simulink subsystem "HV_Battery"  (R2022a)
settings: Solver=VariableStepAuto  StartTime=0.0  StopTime=2474  RelTol=1e-3
model mask{batt_energy=53.5, batt_nominal_voltage=800, coolant_lpm=33.33, coolant_quantity=10, coolant_inlet_temp=25, cell_ambient_temp=35, peak_dischg_c_rate=2, peak_chg_c_rate=2, cont_dischg_c_rate=1, cont_chg_c_rate=1, peak_time=30, peak_time_dischg=0.9, batt_init_soc=0.9}
  mask prompts: batt_energy "Enter the Battery Energy [in kWh]"; batt_nominal_voltage "Enter Battery Nominal Voltage [in V]"; coolant_lpm "Enter Coolant Flow Rate [in LPM]"; coolant_quantity "Enter Coolant Quantity in system [in gallons]"; coolant_inlet_temp "Enter Coolant Initial Inlet Temperature [in Celcius]"; cell_ambient_temp "Enter Local Ambient Cell Temperature [in Celcius]"; peak_dischg_c_rate "Enter Peak Discharge C Rate"; peak_chg_c_rate "Enter Peak Charge C Rate"; cont_dischg_c_rate "Enter Continuous Discharge C Rate"; cont_chg_c_rate "Enter Continuous Charge C Rate"; peak_time "Enter Maximum Duration for Peak Charging C Rate [in seconds]"; peak_time_dischg "Enter Maximum Duration for Peak Discharging C Rate [in seconds]"; batt_init_soc "Enter Initial Battery SOC [0 to 1]"
undefined symbols (not defined in the file or in its folder): batt, cell_Ah, cell_col_eff, cell_cp, cell_eff_area, cell_heat_trans_coeff, cell_mass, cont_chg_current, cont_dischg_current, coolant_cp, coolant_mass, coolant_mass_dot, num_bricks_parallel_in_one_module, num_bricks_series_in_one_module, num_cell_parallel_in_one_brick, num_cell_series_in_one_brick, num_module_Parallel, num_module_Series, peak_chg_current, peak_dischg_current, Total_num_cells
libraries: simulink x18, aerolibconvert2 x3, autolibshared x1
settings Model: DefaultTestHarness=HV_Battery_Harness2  Creator=aak  LastModifiedBy=saumilj

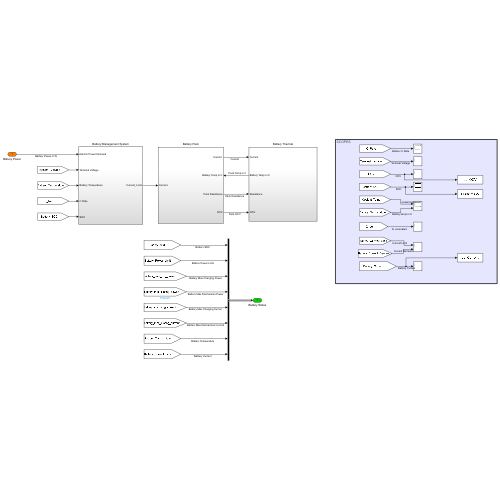
[thumbnail: Simulink's stored preview of the top-level diagram]
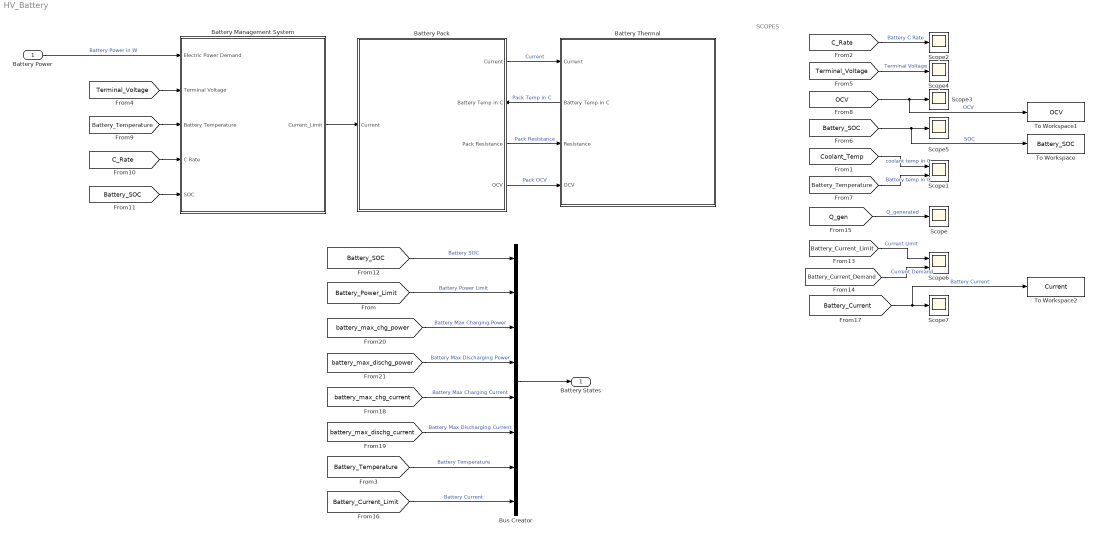
== system HV_Battery ==
  note: SCOPES
  Battery Power : Inport
  Battery Management System : Subsystem
  Battery Pack : Subsystem
      settings: PortSchema="{\"entries\":[{\"content\":{\"sides\":[{\"content\":{\"connectorIds\":[\"In1\"]},\"type\":\"ConnectorPlacement.EquallySpacedRectSide\",\"uuid\":\"b9545a5c-edfc-42ef-81ab-9f23645d84e0\"},{\"content\":{\"connectorIds\":[\"Out1\",\"In2\",\"Out2\",\"Out3\"],\"side\":\"RIGHT\"},\"type\":\"ConnectorPlacement.EquallySpacedRectSide\",\"uuid\":\"40135f2d-ea88-44e9-aecc-89357aa4ea88\"},{\"content\":{\"connectorIds\":[],\"side\":\"TOP\"},\"type\":\"ConnectorPlacement.EquallySpacedRectSide\",\"uuid\":\"2e3e458a-5c5e-47fb-9bfa-05c4f097828d\"},{\"content\":{\"connectorIds\":[],\"side\":\"BOTTOM\"},\"type\":\"ConnectorPlacement.EquallySpacedRectSide\",\"uuid\":\"704f8b5a-b8e4-4dd9-930b-8f21277b1215\"}]},\"type\":\"ConnectorPlacement.EquallySpacedConnector\",\"uuid\":\"37de8f39-e745-4310-bdfe-a8e78e320ee8\"}],\"packageUris\":[\"http://schema.mathworks.com/mf0/Connector/R2020b\"],\"version\":\"1.0\"}"
  Battery Thermal : Subsystem
      settings: PortSchema="{\"entries\":[{\"content\":{\"sides\":[{\"content\":{\"connectorIds\":[\"In1\",\"Out1\",\"In2\",\"In3\"]},\"type\":\"ConnectorPlacement.EquallySpacedRectSide\",\"uuid\":\"af3b2aec-6ad7-445b-b1a0-7265fbd6b2ee\"},{\"content\":{\"connectorIds\":[],\"side\":\"RIGHT\"},\"type\":\"ConnectorPlacement.EquallySpacedRectSide\",\"uuid\":\"a27c7f15-5848-4e0f-a52c-5f856bed419f\"},{\"content\":{\"connectorIds\":[],\"side\":\"TOP\"},\"type\":\"ConnectorPlacement.EquallySpacedRectSide\",\"uuid\":\"1e997449-128f-4f3b-ad87-015e7077aed3\"}]},\"type\":\"ConnectorPlacement.EquallySpacedConnector\",\"uuid\":\"f88aa6e9-d781-4b9c-928f-406822c5ea22\"}],\"packageUris\":[\"http://schema.mathworks.com/mf0/Connector/R2020b\"],\"version\":\"1.0\"}"
  Bus Creator : BusCreator  Inputs=8
  Scope{,2..5,7} (6 alike) : Scope
  Scope1 : Scope  NumInputPorts=2
  Scope6 : Scope  NumInputPorts=2
  To Workspace : ToWorkspace  VariableName=Battery_SOC  SampleTime=-1
  To Workspace1 : ToWorkspace  VariableName=OCV  SampleTime=-1
  To Workspace2 : ToWorkspace  VariableName=Current  SampleTime=-1
  Battery States : Outport
  wires:
  Battery Pack/1("Current ") -> Battery Thermal/1("Current ")  "Current"
  Battery Power/1 -> Battery Management System/1(Electric Power Demand)  "Battery Power in W"
  [Battery_SOC] -> To Workspace/1, Scope5/1  "SOC"
  [OCV] -> To Workspace1/1, Scope3/1  "OCV"
  Battery Thermal/1(Battery Temp in C) -> Battery Pack/2(Battery Temp in C)  "Pack Temp in C"
  [Battery_SOC] -> Battery Management System/5(SOC)
  [Battery_Temperature] -> Scope1/2  "Battery temp in C"
  Battery Management System/1(Current_Limit) -> Battery Pack/1(Current)
  [Terminal_Voltage] -> Battery Management System/2(Terminal Voltage)
  [Battery_SOC] -> Bus Creator/1  "Battery SOC"
  [C_Rate] -> Scope2/1  "Battery C Rate"
  [Battery_Temperature] -> Battery Management System/3(Battery Temperature)
  [Coolant_Temp] -> Scope1/1  "coolant temp in C"
  [Terminal_Voltage] -> Scope4/1  "Terminal Voltage"
  Bus Creator/1 -> Battery States/1
  Battery Pack/2(" Pack Resistance") -> Battery Thermal/2(Resistance)  "Pack Resistance"
  Battery Pack/3(OCV) -> Battery Thermal/3(OCV)  "Pack OCV"
  [C_Rate] -> Battery Management System/4(C Rate)
  [Battery_Power_Limit] -> Bus Creator/2  "Battery Power Limit"
  [Battery_Current_Limit] -> Scope6/1  "Current Limit"
  [Battery_Current_Demand] -> Scope6/2  "Current Demand"
  [Q_gen] -> Scope/1  "Q_generated"
  [Battery_Current] -> To Workspace2/1, Scope7/1  "Battery Current"
  [battery_max_chg_current] -> Bus Creator/5  "Battery Max Charging Current"
  [battery_max_dischg_current] -> Bus Creator/6  "Battery Max Discharging Current"
  [Battery_Temperature] -> Bus Creator/7  "Battery Temperature"
  [Battery_Current_Limit] -> Bus Creator/8  "Battery Current"
  [battery_max_dischg_power] -> Bus Creator/4  "Battery Max Discharging Power"
  [battery_max_chg_power] -> Bus Creator/3  "Battery Max Charging Power"

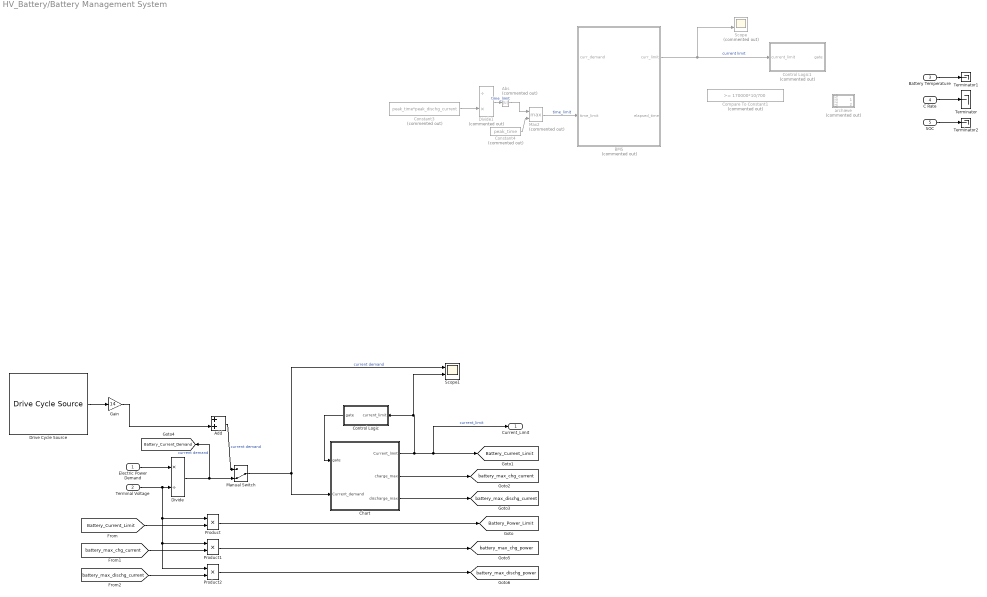
== system HV_Battery/Battery Management System ==
  Electric Power Demand : Inport
  Terminal Voltage : Inport  Port=2
  Battery Temperature : Inport  Port=3
  C Rate : Inport  Port=4
  SOC : Inport  Port=5
  Abs : Abs  Commented=on  SaturateOnIntegerOverflow=off
  Add : Sum
  BMS : Stateflow chart  Commented=on  TreatAsAtomicUnit=on
  Chart : Stateflow chart  TreatAsAtomicUnit=on
      settings: PortSchema="{\"entries\":[{\"content\":{\"sides\":[{\"content\":{\"connectorIds\":[\"In2\",\"In1\"]},\"type\":\"ConnectorPlacement.EquallySpacedRectSide\",\"uuid\":\"61e53cb5-f277-4f3d-99e4-fd5a81de5d3f\"},{\"content\":{\"connectorIds\":[\"Out1\",\"Out2\",\"Out3\"],\"side\":\"RIGHT\"},\"type\":\"ConnectorPlacement.EquallySpacedRectSide\",\"uuid\":\"0e0f51c4-d227-4234-809c-9980418e03b4\"},{\"content\":{\"connectorIds\":[],\"side\":\"TOP\"},\"type\":\"ConnectorPlacement.EquallySpacedRectSide\",\"uuid\":\"31baac4d-e034-4979-aab1-cd5457b5efab\"}]},\"type\":\"ConnectorPlacement.EquallySpacedConnector\",\"uuid\":\"6907569d-9725-4403-be47-b0224ef335f3\"}],\"packageUris\":[\"http://schema.mathworks.com/mf0/Connector/R2020b\"],\"version\":\"1.0\"}"
  Compare To Constant1 : simulink/Logic and Bit Operations/Compare To Constant  Commented=on  relop=>=  const=170000*10/700  OutDataTypeStr=boolean
  Constant3 : Constant  Commented=on  Value=peak_time*peak_dischg_current
  Constant4 : Constant  Commented=on  Value=peak_time
  Control Logic : Subsystem
      settings: PortSchema="{\"entries\":[{\"content\":{\"sides\":[{\"content\":{\"connectorIds\":[\"Out1\"]},\"type\":\"ConnectorPlacement.EquallySpacedRectSide\",\"uuid\":\"375a58bc-16a4-4cbe-8416-d0abc0116f23\"},{\"content\":{\"connectorIds\":[\"In1\"],\"side\":\"RIGHT\"},\"type\":\"ConnectorPlacement.EquallySpacedRectSide\",\"uuid\":\"b00af4b7-7940-47c4-950c-bf6d404947a6\"},{\"content\":{\"connectorIds\":[],\"side\":\"TOP\"},\"type\":\"ConnectorPlacement.EquallySpacedRectSide\",\"uuid\":\"5f8d3327-63b2-477e-9ddb-4def616de5d9\"}]},\"type\":\"ConnectorPlacement.EquallySpacedConnector\",\"uuid\":\"dfdcbaa4-409c-473f-908d-88d904123078\"}],\"packageUris\":[\"http://schema.mathworks.com/mf0/Connector/R2020b\"],\"version\":\"1.0\"}"
  Control Logic1 : Subsystem  Commented=on
  Divide : Product  Inputs=*/
  Divide1 : Product  Commented=on  Inputs=/*
  Drive Cycle Source : autolibshared/Drive Cycle Source  cycleVar=FTP75  fileVar=cycleFTP75.mat  tfinal="2474  seconds, Cyclic"  cycleRepeat=on  outAccPort=off  outGearPort=off  gearList=No gear data  t_wot1=5  xdot_woto=0  xdot_wot1=30  t_wot2=20  xdot_wot2=0  t_wotend=30  srcUnit=m/s  outUnit=m/s  srcAccUnit=m/s/s  outAccUnit=m/s^2  dt=1  aMode=1  faultOption=off  velBnd=2  velBndUnit=mph  inUnit=m/s  timeBnd=1  failOption=off  stopSim=off  maxFaultCnt=10  maxFaultTime=2  maxTotFaultTime=15  traceOption=off  dtTrace=1  traceWindow=10  lastDCname=FTP75  lastOutUnit=mph  lastDT=1  lastTB=1  lastSB=2  forceCalcBound=off
      settings: SourceProductBaseCode=PW,DR,MT,VE
  Gain : Gain  Gain=14
  Manual Switch : ManualSwitch  CurrentSetting=0
  Max2 : MinMax  Commented=on  Function=max  Inputs=2
  Product : Product
  Product1 : Product
  Product2 : Product
  Scope : Scope  Commented=on  NumInputPorts=2
  Scope1 : Scope  NumInputPorts=2
  Terminator : Terminator
  Terminator1 : Terminator
  Terminator2 : Terminator
  archieve : Subsystem  Commented=on
  Current_Limit : Outport
  tag scope: Battery_Current_Demand=global, Battery_Current_Limit=global, Battery_Power_Limit=global, battery_max_chg_current=global, battery_max_chg_power=global, battery_max_dischg_current=global, battery_max_dischg_power=global
  wires:
  [battery_max_dischg_current] -> Product2/2
  Product2/1 -> [battery_max_dischg_power]
  Product1/1 -> [battery_max_chg_power]
  [battery_max_chg_current] -> Product1/2
  Control Logic/1(gate) -> Chart/2(gate)
  Electric Power Demand/1 -> Divide/1
  Drive Cycle Source/1 -> Gain/1
  Product/1 -> [Battery_Power_Limit]
  [Battery_Current_Limit] -> Product/2
  Manual Switch/1 -> Chart/1(Current_demand), Scope1/1  "current demand"
  Add/1 -> Manual Switch/1  "current demand"
  Gain/1 -> Add/2
  Chart/1(Current_limit) -> Scope1/2, Control Logic/1(current_limit), Current_Limit/1, [Battery_Current_Limit]  "current_limit"
  BMS/1(curr_limit) -> Control Logic1/1(current_limit), Scope/2  "current limit"
  Abs/1 -> Max2/1
  Constant4/1 -> Max2/2
  Max2/1 -> BMS/2(time_limit)  "time_limit"
  Divide/1 -> Manual Switch/2, [Battery_Current_Demand]  "current demand"
  Terminal Voltage/1 -> Divide/2, Product/1, Product1/1, Product2/1
  C Rate/1 -> Terminator/1
  Battery Temperature/1 -> Terminator1/1
  SOC/1 -> Terminator2/1
  Divide1/1 -> Abs/1  "time_limit"
  Constant3/1 -> Divide1/2
  Chart/2(charge_max) -> [battery_max_chg_current]
  Chart/3(discharge_max) -> [battery_max_dischg_current]

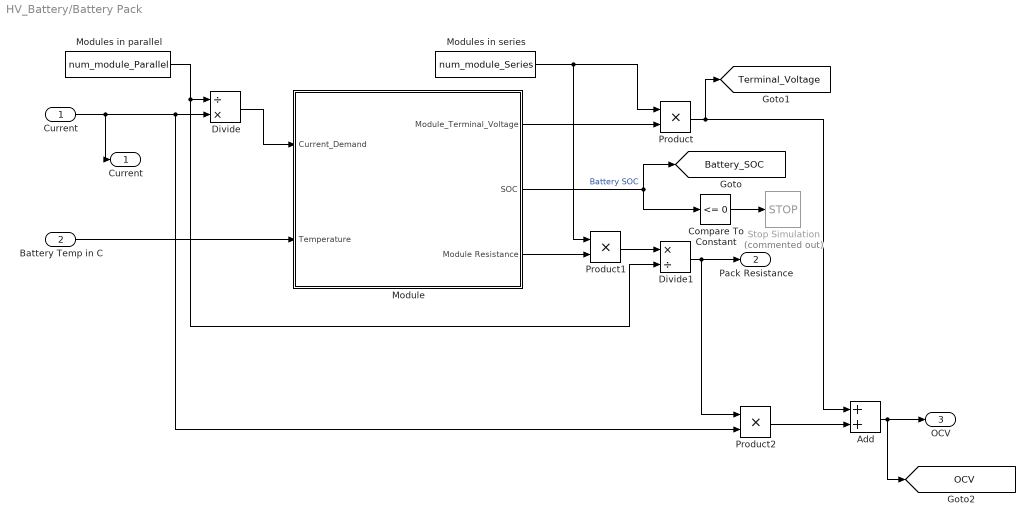
== system HV_Battery/Battery Pack ==
  Current : Inport
  Battery Temp in C : Inport  Port=2
  Add : Sum
  Compare To Constant : simulink/Logic and Bit Operations/Compare To Constant  relop=<=  const=0  OutDataTypeStr=boolean
  Divide : Product  Inputs=/*
  Divide1 : Product  Inputs=*/
  Module : Subsystem
  Modules in parallel : Constant  Value=num_module_Parallel
  Modules in series : Constant  Value=num_module_Series
  Product : Product
  Product1 : Product
  Product2 : Product
  Stop Simulation : Stop  Commented=on
  "Current " : Outport
  " Pack Resistance" : Outport  Port=2
  OCV : Outport  Port=3
  tag scope: Battery_SOC=global, OCV=global, Terminal_Voltage=global
  wires:
  Module/2(" SOC") -> Compare To Constant/1, [Battery_SOC]  "Battery SOC"
  Compare To Constant/1 -> Stop Simulation/1
  Divide/1 -> Module/1(Current_Demand)
  Module/1(Module_Terminal_Voltage) -> Product/2
  Product/1 -> [Terminal_Voltage], Add/1
  Divide1/1 -> Product2/1, " Pack Resistance"/1
  Modules in series/1 -> Product/1, Product1/1
  Product1/1 -> Divide1/1
  Module/3(" Module Resistance") -> Product1/2
  Modules in parallel/1 -> Divide/1, Divide1/2
  Battery Temp in C/1 -> Module/2(Temperature)
  Product2/1 -> Add/2
  Add/1 -> OCV/1, [OCV]
  Current/1 -> Product2/2, Divide/2, "Current "/1

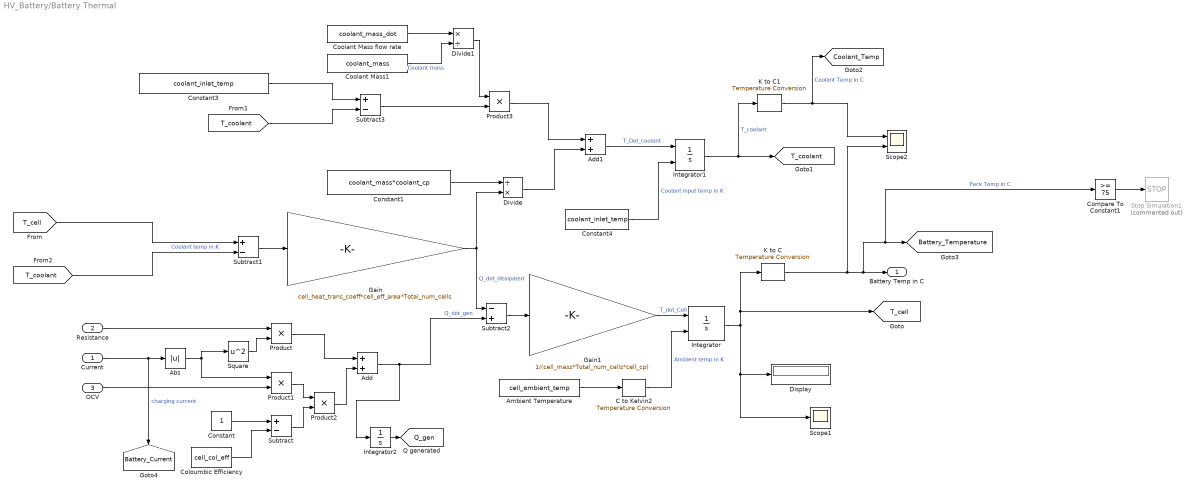
== system HV_Battery/Battery Thermal ==
  "Current " : Inport
  Resistance : Inport  Port=2
  OCV : Inport  Port=3
  Abs : Abs  SaturateOnIntegerOverflow=off
  Add : Sum
  Add1 : Sum
  Ambient Temperature : Constant  Value=cell_ambient_temp
  C to Kelvin2 : aerolibconvert2/Temperature Conversion  IU=C  OU=K
      settings: SourceProductBaseCode=AE
  Coloumbic Efficiency : Constant  Value=cell_col_eff
  Compare To Constant1 : simulink/Logic and Bit Operations/Compare To Constant  relop=>=  const=75  OutDataTypeStr=boolean
  Constant : Constant
  Constant1 : Constant  Value=coolant_mass*coolant_cp
  Constant3 : Constant  Value=coolant_inlet_temp
  Constant4 : Constant  Value=coolant_inlet_temp
  Coolant Mass flow rate : Constant  Value=coolant_mass_dot
  Coolant Mass1 : Constant  Value=coolant_mass
  Display : Display
  Divide : Product  Inputs=/*
  Divide1 : Product  Inputs=*/
  Gain : Gain  Gain=cell_heat_trans_coeff*cell_eff_area*Total_num_cells
  Gain1 : Gain  Gain=1/(cell_mass*Total_num_cells*cell_cp)
  Integrator : Integrator  InitialConditionSource=external  InitialCondition=273+25
  Integrator1 : Integrator  InitialConditionSource=external
  Integrator2 : Integrator
  K to C : aerolibconvert2/Temperature Conversion  IU=K  OU=C
      settings: SourceProductBaseCode=AE
  K to C1 : aerolibconvert2/Temperature Conversion  IU=K  OU=C
      settings: SourceProductBaseCode=AE
  Product{,1..3} (4 alike) : Product
  Scope1 : Scope
  Scope2 : Scope  NumInputPorts=2
  Square : Math  Operator=square
  Stop Simulation1 : Stop  Commented=on
  Subtract : Sum  Inputs=+-
  Subtract1 : Sum  Inputs=+-
  Subtract2 : Sum  Inputs=-+
  Subtract3 : Sum  Inputs=+-
  Battery Temp in C : Outport
  tag scope: Battery_Current=global, Battery_Temperature=global, Coolant_Temp=global, Q_gen=global, T_cell=global, T_coolant=global
  wires:
  K to C/1 -> Scope2/2, Battery Temp in C/1, [Battery_Temperature], Compare To Constant1/1  "Pack Temp in C"
  Compare To Constant1/1 -> Stop Simulation1/1
  Resistance/1 -> Product/1
  Square/1 -> Product/2
  OCV/1 -> Product1/2
  Constant/1 -> Subtract/1
  Coloumbic Efficiency/1 -> Subtract/2
  Product1/1 -> Product2/1
  Subtract/1 -> Product2/2
  Product/1 -> Add/1
  Product2/1 -> Add/2
  Add/1 -> Integrator2/1, Subtract2/2  "Q_dot_gen"
  [T_coolant] -> Subtract1/2  "Coolant temp in K"
  Subtract1/1 -> Gain/1
  Gain1/1 -> Integrator/1  "T_dot_Cell"
  Integrator/1 -> Display/1, Scope1/1, K to C/1, [T_cell]
  [T_cell] -> Subtract1/1
  Subtract2/1 -> Gain1/1
  Gain/1 -> Subtract2/1, Divide/2  "Q_dot_dissipated"
  Ambient Temperature/1 -> C to Kelvin2/1
  C to Kelvin2/1 -> Integrator/2  "Ambient temp in K"
  Constant1/1 -> Divide/1
  Divide/1 -> Add1/2
  Constant3/1 -> Subtract3/1
  [T_coolant] -> Subtract3/2
  Subtract3/1 -> Product3/2
  Product3/1 -> Add1/1
  Add1/1 -> Integrator1/1  "T_Dot_coolant"
  Integrator1/1 -> K to C1/1, [T_coolant]  "T_coolant"
  "Current "/1 -> [Battery_Current], Abs/1  "charging current"
  Coolant Mass flow rate/1 -> Divide1/1
  Divide1/1 -> Product3/1
  Coolant Mass1/1 -> Divide1/2  "Coolant mass"
  Constant4/1 -> Integrator1/2  "Coolant input temp in K"
  K to C1/1 -> [Coolant_Temp], Scope2/1  "Coolant Temp in C"
  Abs/1 -> Square/1, Product1/1
  Integrator2/1 -> [Q_gen]

== system HV_Battery/Battery Management System/Control Logic ==
  current_limit : Inport
  Charging : Subsystem
  Discharging : Subsystem
  Switch : Switch  Criteria=u2 > Threshold  SaturateOnIntegerOverflow=off  InputSameDT=off
  gate : Outport
  wires:
  current_limit/1 -> Discharging/1(current limit), Switch/2, Charging/1(current limit)
  Charging/1(charging gate) -> Switch/3, gate/1
  Discharging/1(discharging gate) -> Switch/1

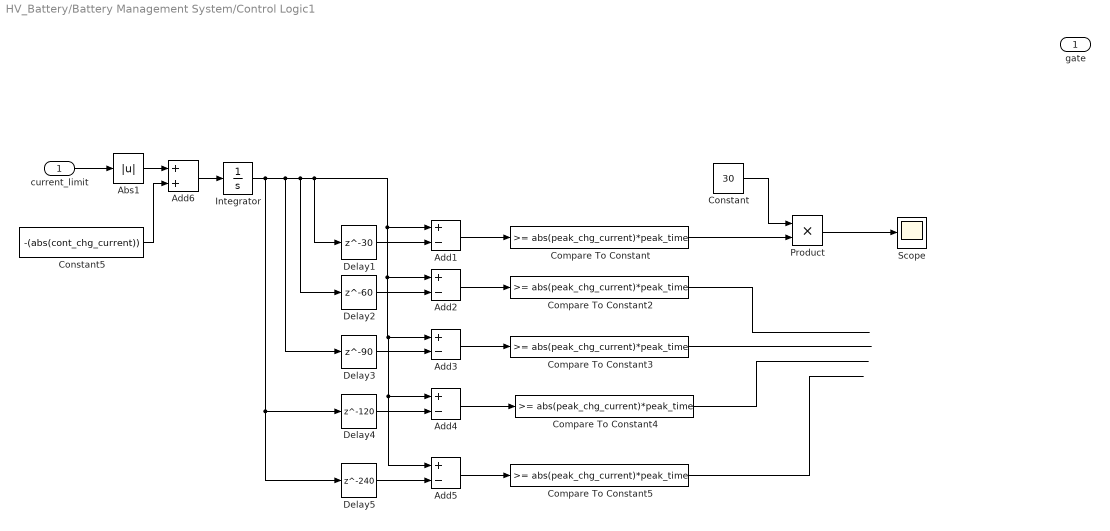
== system HV_Battery/Battery Management System/Control Logic1 ==
  current_limit : Inport
  Abs1 : Abs  SaturateOnIntegerOverflow=off
  Add{1..5} (5 alike) : Sum  Inputs=+-
  Add6 : Sum
  Compare To Constant{,2..5} (5 alike) : simulink/Logic and Bit Operations/Compare To Constant  relop=>=  const=abs(peak_chg_current)*peak_time  OutDataTypeStr=boolean
  Constant : Constant  Value=30
  Constant5 : Constant  Value=-(abs(cont_chg_current))
  Delay1 : Delay  DelayLength=30  SampleTime=1
  Delay2 : Delay  DelayLength=60  SampleTime=1
  Delay3 : Delay  DelayLength=90  SampleTime=1
  Delay4 : Delay  DelayLength=120  SampleTime=1
  Delay5 : Delay  DelayLength=240  SampleTime=1
  Integrator : Integrator  LimitOutput=on  LowerSaturationLimit=0
  Product : Product
  Scope : Scope
  gate : Outport
  wires:
  ? -> gate/1
  Add4/1 -> Compare To Constant4/1
  Add1/1 -> Compare To Constant/1
  Delay4/1 -> Add4/2
  Add2/1 -> Compare To Constant2/1
  Delay3/1 -> Add3/2
  Compare To Constant5/1 -> ?
  Compare To Constant4/1 -> ?
  Abs1/1 -> Add6/1
  Add3/1 -> Compare To Constant3/1
  Add6/1 -> Integrator/1
  Delay5/1 -> Add5/2
  Delay2/1 -> Add2/2
  Compare To Constant2/1 -> ?
  Constant5/1 -> Add6/2
  Compare To Constant3/1 -> ?
  Integrator/1 -> Delay4/1, Delay5/1, Add1/1, Add2/1, Add3/1, Add4/1, Add5/1, Delay1/1, Delay2/1, Delay3/1
  Delay1/1 -> Add1/2
  Add5/1 -> Compare To Constant5/1
  current_limit/1 -> Abs1/1
  Constant/1 -> Product/1
  Compare To Constant/1 -> Product/2
  Product/1 -> Scope/1

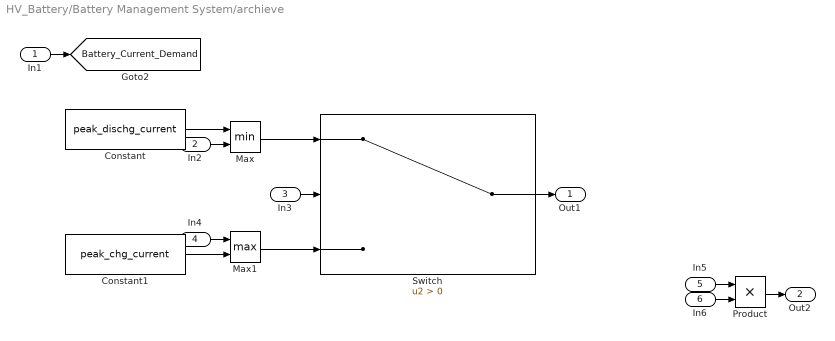
== system HV_Battery/Battery Management System/archieve ==
  In1 : Inport
  In2 : Inport  Port=2
  In3 : Inport  Port=3
  In4 : Inport  Port=4
  In5 : Inport  Port=5
  In6 : Inport  Port=6
  Constant : Constant  Value=peak_dischg_current
  Constant1 : Constant  Value=peak_chg_current
  Max : MinMax  Inputs=2
  Max1 : MinMax  Function=max  Inputs=2
  Product : Product
  Switch : Switch  Criteria=u2 > Threshold  SaturateOnIntegerOverflow=off  InputSameDT=off
  Out1 : Outport
  Out2 : Outport  Port=2
  tag scope: Battery_Current_Demand=global
  wires:
  In4/1 -> Max1/1
  Product/1 -> Out2/1
  In3/1 -> Switch/2
  Switch/1 -> Out1/1
  In2/1 -> Max/2
  In6/1 -> Product/2
  Constant1/1 -> Max1/2
  In5/1 -> Product/1
  Constant/1 -> Max/1
  Max/1 -> Switch/1
  Max1/1 -> Switch/3
  In1/1 -> [Battery_Current_Demand]

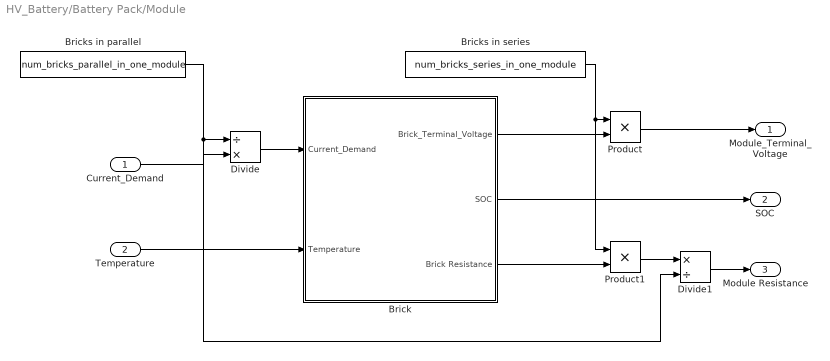
== system HV_Battery/Battery Pack/Module ==
  Current_Demand : Inport
  Temperature : Inport  Port=2
  Brick : Subsystem
  Bricks in parallel : Constant  Value=num_bricks_parallel_in_one_module
  Bricks in series : Constant  Value=num_bricks_series_in_one_module
  Divide : Product  Inputs=/*
  Divide1 : Product  Inputs=*/
  Product : Product
  Product1 : Product
  Module_Terminal_Voltage : Outport
  " SOC" : Outport  Port=2
  " Module Resistance" : Outport  Port=3
  wires:
  Current_Demand/1 -> Divide/2
  Divide/1 -> Brick/1(Current_Demand)
  Brick/1(Brick_Terminal_Voltage) -> Product/2
  Product/1 -> Module_Terminal_Voltage/1
  Brick/2(" SOC") -> " SOC"/1
  Temperature/1 -> Brick/2(Temperature)
  Bricks in parallel/1 -> Divide/1, Divide1/2
  Product1/1 -> Divide1/1
  Divide1/1 -> " Module Resistance"/1
  Bricks in series/1 -> Product1/1, Product/1
  Brick/3(" Brick Resistance") -> Product1/2

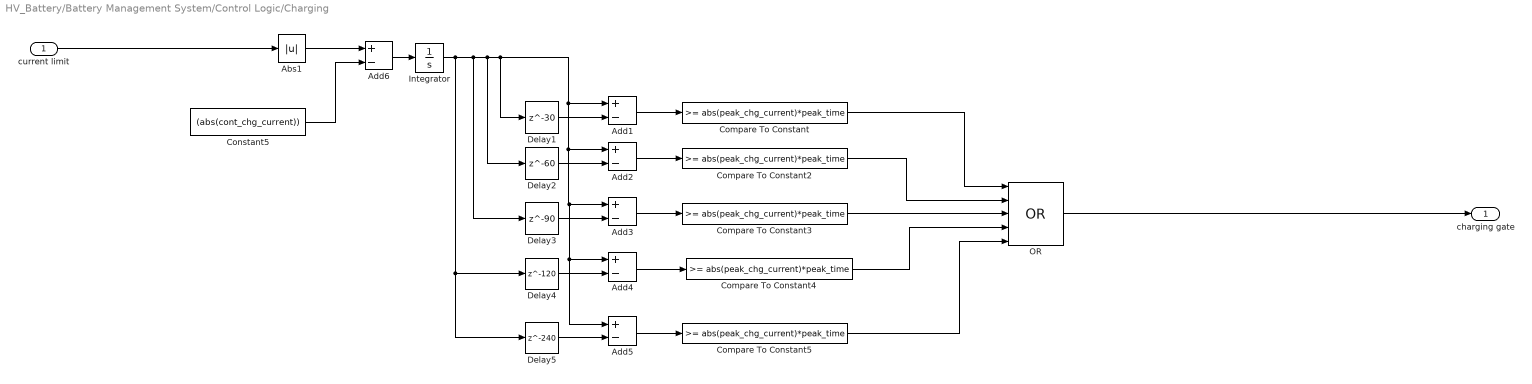
== system HV_Battery/Battery Management System/Control Logic/Charging ==
  current limit : Inport
  Abs1 : Abs  SaturateOnIntegerOverflow=off
  Add{1..6} (6 alike) : Sum  Inputs=+-
  Compare To Constant{,2..5} (5 alike) : simulink/Logic and Bit Operations/Compare To Constant  relop=>=  const=abs(peak_chg_current)*peak_time  OutDataTypeStr=boolean
  Constant5 : Constant  Value=(abs(cont_chg_current))
  Delay1 : Delay  DelayLength=30  SampleTime=1
  Delay2 : Delay  DelayLength=60  SampleTime=1
  Delay3 : Delay  DelayLength=90  SampleTime=1
  Delay4 : Delay  DelayLength=120  SampleTime=1
  Delay5 : Delay  DelayLength=240  SampleTime=1
  Integrator : Integrator  LimitOutput=on  LowerSaturationLimit=0
  OR : Logic  Operator=OR  Inputs=5  IconShape=distinctive  AllPortsSameDT=off  OutDataTypeStr=boolean
  charging gate : Outport
  wires:
  Add4/1 -> Compare To Constant4/1
  Constant5/1 -> Add6/2
  Add1/1 -> Compare To Constant/1
  OR/1 -> charging gate/1
  Add6/1 -> Integrator/1
  Compare To Constant5/1 -> OR/5
  Compare To Constant4/1 -> OR/4
  Delay2/1 -> Add2/2
  Integrator/1 -> Delay4/1, Delay5/1, Add1/1, Add2/1, Add3/1, Add4/1, Add5/1, Delay1/1, Delay2/1, Delay3/1
  Delay4/1 -> Add4/2
  Abs1/1 -> Add6/1
  Add2/1 -> Compare To Constant2/1
  Delay3/1 -> Add3/2
  Delay5/1 -> Add5/2
  Add5/1 -> Compare To Constant5/1
  Delay1/1 -> Add1/2
  current limit/1 -> Abs1/1
  Compare To Constant3/1 -> OR/3
  Add3/1 -> Compare To Constant3/1
  Compare To Constant/1 -> OR/1
  Compare To Constant2/1 -> OR/2

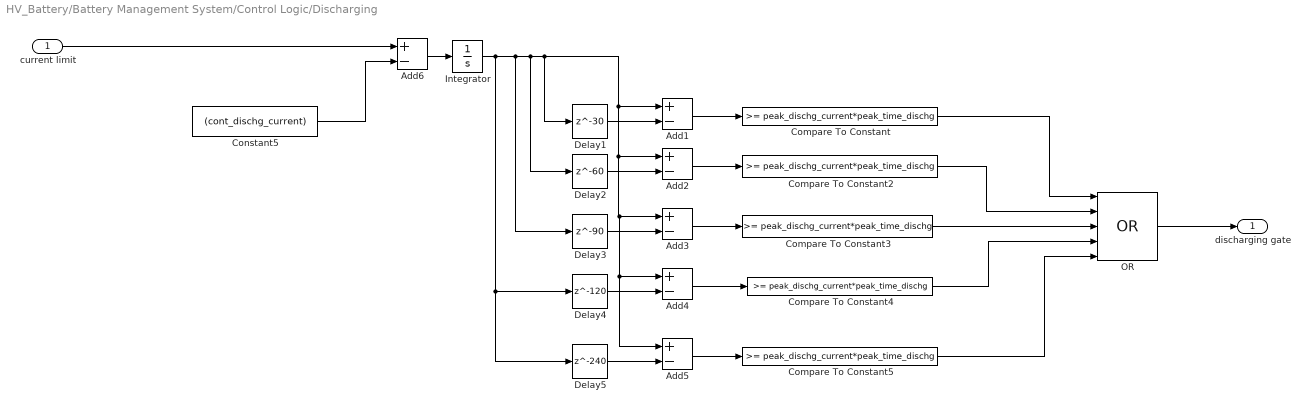
== system HV_Battery/Battery Management System/Control Logic/Discharging ==
  current limit : Inport
  Add{1..6} (6 alike) : Sum  Inputs=+-
  Compare To Constant{,2..5} (5 alike) : simulink/Logic and Bit Operations/Compare To Constant  relop=>=  const=peak_dischg_current*peak_time_dischg  OutDataTypeStr=boolean
  Constant5 : Constant  Value=(cont_dischg_current)
  Delay1 : Delay  DelayLength=30  SampleTime=1
  Delay2 : Delay  DelayLength=60  SampleTime=1
  Delay3 : Delay  DelayLength=90  SampleTime=1
  Delay4 : Delay  DelayLength=120  SampleTime=1
  Delay5 : Delay  DelayLength=240  SampleTime=1
  Integrator : Integrator  LimitOutput=on  LowerSaturationLimit=0
  OR : Logic  Operator=OR  Inputs=5  IconShape=distinctive  AllPortsSameDT=off  OutDataTypeStr=boolean
  discharging gate : Outport
  wires:
  Add4/1 -> Compare To Constant4/1
  Constant5/1 -> Add6/2
  Add1/1 -> Compare To Constant/1
  OR/1 -> discharging gate/1
  Add6/1 -> Integrator/1
  Compare To Constant5/1 -> OR/5
  Compare To Constant4/1 -> OR/4
  Delay2/1 -> Add2/2
  Integrator/1 -> Delay4/1, Delay5/1, Add1/1, Add2/1, Add3/1, Add4/1, Add5/1, Delay1/1, Delay2/1, Delay3/1
  Delay4/1 -> Add4/2
  current limit/1 -> Add6/1
  Add2/1 -> Compare To Constant2/1
  Delay3/1 -> Add3/2
  Delay5/1 -> Add5/2
  Add5/1 -> Compare To Constant5/1
  Delay1/1 -> Add1/2
  Compare To Constant3/1 -> OR/3
  Add3/1 -> Compare To Constant3/1
  Compare To Constant/1 -> OR/1
  Compare To Constant2/1 -> OR/2

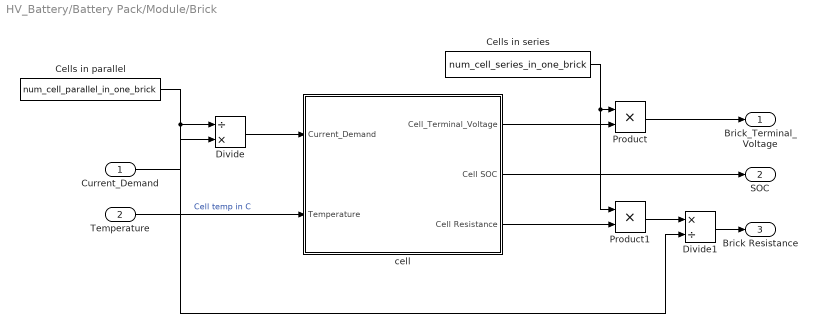
== system HV_Battery/Battery Pack/Module/Brick ==
  Current_Demand : Inport
  Temperature : Inport  Port=2
  Cells in parallel : Constant  Value=num_cell_parallel_in_one_brick
  Cells in series : Constant  Value=num_cell_series_in_one_brick
  Divide : Product  Inputs=/*
  Divide1 : Product  Inputs=*/
  Product : Product
  Product1 : Product
  cell : Subsystem
  Brick_Terminal_Voltage : Outport
  " SOC" : Outport  Port=2
  " Brick Resistance" : Outport  Port=3
  wires:
  Current_Demand/1 -> Divide/2
  Divide/1 -> cell/1(Current_Demand)
  Cells in series/1 -> Product1/1, Product/1
  Product/1 -> Brick_Terminal_Voltage/1
  cell/1(Cell_Terminal_Voltage) -> Product/2
  cell/2(Cell SOC) -> " SOC"/1
  Temperature/1 -> cell/2(Temperature)  "Cell temp in C"
  cell/3(Cell Resistance) -> Product1/2
  Product1/1 -> Divide1/1
  Cells in parallel/1 -> Divide/1, Divide1/2
  Divide1/1 -> " Brick Resistance"/1

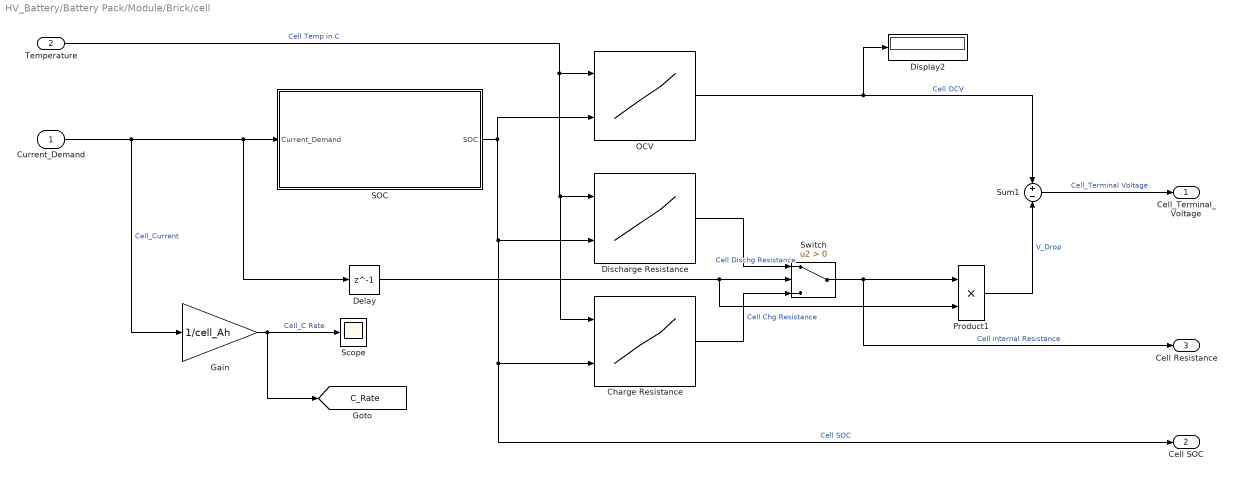
== system HV_Battery/Battery Pack/Module/Brick/cell ==
  Current_Demand : Inport
  Temperature : Inport  Port=2
  Charge Resistance : Lookup_n-D  BreakpointsForDimension1=batt.res.temp  BreakpointsForDimension2=batt.res.soc  Table=batt.res.chg  InternalRulePriority=Speed  RndMeth=Simplest
      settings: InputPortMap=u0,u1
  Delay : Delay  DelayLength=1
  Discharge Resistance : Lookup_n-D  BreakpointsForDimension1=batt.res.temp  BreakpointsForDimension2=batt.res.soc  Table=batt.res.dischg  InternalRulePriority=Speed  RndMeth=Simplest
      settings: InputPortMap=u0,u1
  Display2 : Display
  Gain : Gain  Gain=1/cell_Ah
  OCV : Lookup_n-D  BreakpointsForDimension1=batt.res.temp  BreakpointsForDimension2=batt.res.soc  Table=batt.ocv.ocv  InternalRulePriority=Speed  RndMeth=Simplest
      settings: InputPortMap=u0,u1
  Product1 : Product
  SOC : Subsystem
  Scope : Scope
  Sum1 : Sum  Inputs=+-
  Switch : Switch  Criteria=u2 > Threshold  SaturateOnIntegerOverflow=off  InputSameDT=off
  Cell_Terminal_Voltage : Outport
  Cell SOC : Outport  Port=2
  Cell Resistance : Outport  Port=3
  tag scope: C_Rate=global
  wires:
  Temperature/1 -> Charge Resistance/1, Discharge Resistance/1, OCV/1  "Cell Temp in C"
  OCV/1 -> Sum1/1, Display2/1  "Cell OCV"
  SOC/1(SOC) -> OCV/2, Cell SOC/1, Charge Resistance/2, Discharge Resistance/2  "Cell SOC"
  Charge Resistance/1 -> Switch/3  "Cell Chg Resistance"
  Discharge Resistance/1 -> Switch/1  "Cell Dischg Resistance"
  Current_Demand/1 -> Gain/1, Delay/1, SOC/1(Current_Demand)  "Cell_Current"
  Switch/1 -> Cell Resistance/1, Product1/1  "Cell internal Resistance"
  Product1/1 -> Sum1/2  "V_Drop"
  Sum1/1 -> Cell_Terminal_Voltage/1  "Cell_Terminal Voltage"
  Delay/1 -> Product1/2, Switch/2
  Gain/1 -> [C_Rate], Scope/1  "Cell_C Rate"

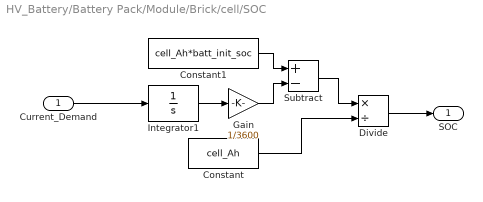
== system HV_Battery/Battery Pack/Module/Brick/cell/SOC ==
  Current_Demand : Inport
  Constant : Constant  Value=cell_Ah
  Constant1 : Constant  Value=cell_Ah*batt_init_soc
  Divide : Product  Inputs=*/
  Gain : Gain  Gain=1/3600
  Integrator1 : Integrator
  Subtract : Sum  Inputs=+-
  SOC : Outport
  wires:
  Current_Demand/1 -> Integrator1/1
  Integrator1/1 -> Gain/1
  Constant/1 -> Divide/2
  Divide/1 -> SOC/1
  Constant1/1 -> Subtract/1
  Gain/1 -> Subtract/2
  Subtract/1 -> Divide/1

== stateflow chart HV_Battery/Battery Management System/Chart ==
  state state_0
    du:
    Current_limit = max(peak_chg_current,min(peak_dischg_current,Current_demand));
    discharge_max = peak_dischg_current;
    charge_max = peak_chg_current;
  state state_1
    du:
    Current_limit = max(cont_chg_current,min(cont_dischg_current,Current_demand));
    discharge_max = cont_dischg_current;
    charge_max = cont_chg_current;
  (default) -> state_0
  state_0 -> state_1 : [gate == 1]
  state_1 -> state_0 : [gate==0]
  data: Current_demand input; gate input; Current_limit output; cont_dischg_current parameter; peak_dischg_current parameter double; peak_chg_current parameter; charge_max output; discharge_max output; cont_chg_current parameter

== stateflow chart HV_Battery/Battery Management System/BMS ==
  state Discharge
    state Continuous
      du:
      curr_limit = min(cont_dischg_current,curr_demand);
    state Peak
      du:
      curr_limit = min(curr_demand,peak_dischg_current);
      elapsed_time = elapsed(sec);
    (default) -> Discharge.Continuous : {a=0;b=0;elapsed_time=0;t=0;}
    Discharge.Continuous -> Discharge.Peak : [((curr_demand > cont_dischg_current) && a ==1 && after(((t/2)),sec) ) || ((curr_demand > cont_dischg_current) && b ==0)]{elapsed_time = 0;}
    Discharge.Peak -> Discharge.Continuous : [after(((time_limit)),sec) || (curr_demand <= cont_dischg_current)]{a=1;b=1;elapsed_time = 0;t=time_limit;}
  state Charge
    state Continuous
      du:
      curr_limit = max(cont_chg_current,curr_demand);
    state Peak
      du:
      curr_limit = max(curr_demand,peak_chg_current);
    (default) -> Charge.Continuous : {a=0;b=0}
    Charge.Continuous -> Charge.Peak : [((abs(curr_demand) > abs(cont_chg_current)) && a ==1 &&  after((time_limit/2),sec) ) || ((abs(curr_demand) > abs(cont_chg_current)) && b ==0)]
  (default) -> Discharge
  Discharge -> Charge : [curr_demand < 0]
  Charge -> Discharge : [curr_demand >= 0]
  data: curr_demand input; curr_limit output; peak_dischg_current parameter double; peak_chg_current parameter double; cont_chg_current parameter; cont_dischg_current parameter; a local; b local; time_limit input; elapsed_time output; t local
